simulink model "Preprocesado2"  (R2021b)
settings: Solver=VariableStepAuto  StartTime=0.0  StopTime=1  RelTol=1e-3
undefined symbols (not defined in the file): fdesignblkfcn, gcbh
libraries: dsparch4 x1
settings Model: Creator=alvaro  LastModifiedBy=alvaro

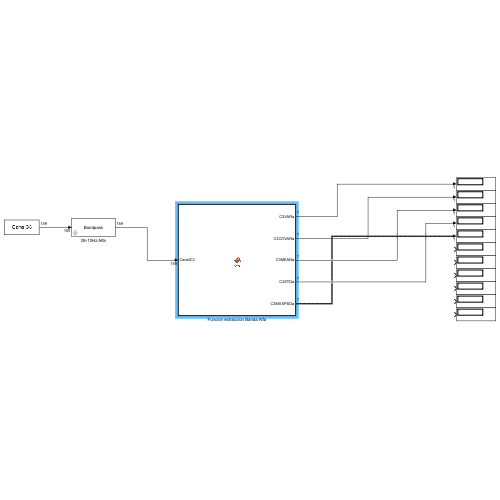
[thumbnail: Simulink's stored preview of the top-level diagram]
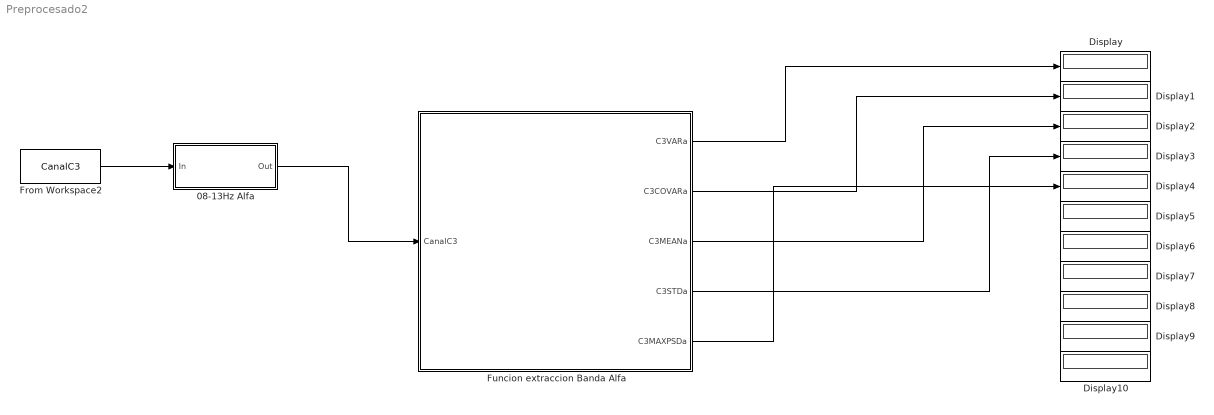
== system Preprocesado2 ==
  08-13Hz Alfa : Subsystem  DialogController=fdesignblkfcn  InitFcn=fdesignblkfcn(gcbh, {'InitFcn'});  mask(Bandpass Filter){}
      mask help: Design a bandpass filter
      settings: CopyFcn=fdesignblkfcn(gcbh, {'CopyFcn'});
      mask Help: helpview(mapfilelocation('dsp'), 'dspbandpassfilter');
      mask Display: disp('Bandpass');
  Display{,1..10} (11 alike) : Display
  From Workspace2 : FromWorkspace  VariableName=CanalC3  SampleTime=160
  Funcion extraccion Banda Alfa : MATLAB Function  TreatAsAtomicUnit=on
  wires:
  Funcion extraccion Banda Alfa/1(C3VARa) -> Display/1
  From Workspace2/1 -> 08-13Hz Alfa/1(In)
  08-13Hz Alfa/1(Out) -> Funcion extraccion Banda Alfa/1(CanalC3)
  Funcion extraccion Banda Alfa/2(C3COVARa) -> Display1/1
  Funcion extraccion Banda Alfa/3(C3MEANa) -> Display2/1
  Funcion extraccion Banda Alfa/4(C3STDa) -> Display3/1
  Funcion extraccion Banda Alfa/5(C3MAXPSDa) -> Display4/1

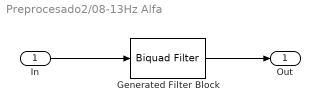
== system Preprocesado2/08-13Hz Alfa ==
  In : Inport
  Generated Filter Block : dsparch4/Biquad Filter  Tag=BlockMethodSubSystem  FilterSource=Dialog parameters  CoeffSource=Specify via dialog  FilterObject=BQF  IIRFiltStruct=Direct form II  BiQuadCoeffs=[0.106193777977083598 0 -0.106193777977083598 1 -1.70817022912376837 0.836223107513699437;0.0287712784311114321 0 -0.0287712784311114321 1 -1.65259216844571899 0.816617541167721783;0.228933752509714789 0 -0.228933752509714789 1 -1.86379720464038678 0.961272776502518855;0.0557488790708176307 0 -0.0557488790708176307 1 -1.69650707415507318 0.940282353609846799;0.182028469565088447 0 -0.182028469565088447 1 -1.7845677565195861 0.890495241818041738;1.50270841788426179 0 -1.50270841788426179 1 -1.64361878317248067 0.850702967185112069]  ScaleValues=[0.0585193363851460036;1;1;1;1;1;1]  IC=0  ICnum=0  ICden=0  a0Flag=Warning  optimizeScaleValues=on  ScaleValueMode=Specify via input port (g)  roundingMode=Floor  overflowMode=off  scaleValueFracLength=14  denProdOutputFracLength=30  denAccumFracLength=30  secondMemoryFracLength=15
  Out : Outport
  wires:
  In/1 -> Generated Filter Block/1
  Generated Filter Block/1 -> Out/1

== matlab function Preprocesado2/Funcion extraccion Banda Alfa ==
  settings: updateMethod=DISCRETE  sampleTime=160
  data: C3VARa output; CanalC3 input; C3COVARa output; C3MEANa output; C3STDa output [1..999999]; C3MAXPSDa output
function [C3VARa,C3COVARa, C3MEANa, C3STDa, C3MAXPSDa] = fcn(CanalC3)
c3alfat=CanalC3;

%Funcion Wavalet para descomponer la señas y tener reducir el nº de muestras
[cc3 ,lc3]= wavedec(c3alfat,2,'db2');
c3alfat = appcoef(cc3,lc3,'db2'); 

%Calculamos la Densidad espectral de Potencia mediante el metodo Welch 
[C3welchalfa,f] = pwelch(c3alfat);
f=(f/2*pi)*80;
%Calculamos la FFT de la señal.
C3alfat = abs(fft(c3alfat)); 

%%Extracion de Caracteristicas 
% Alfa 
C3VARa=var(C3alfat);
C3COVARa=cov(C3alfat);
C3MEANa=mean(C3alfat);
C3STDa=std(C3alfat);
C3MAXPSDa=max(C3welchalfa);
c3VARa=var(c3alfat);
c3COVARa=cov(c3alfat);
c3MEANa=cov(c3alfat);
c3STDa=std(c3alfat);
c3MAXa=max(c3alfat);
c3MINa=min(c3alfat);
